simulink model "RobotStepID"  (R2022b)
settings: Solver=VariableStepAuto  StartTime=0.0  StopTime=10.0  RelTol=1e-3
values from neighbouring files (symbols this model uses):
  kPhi = 3.3*12.5    (= 41.25)    [demo1_avgVa_Identification.m]    (also in robotContVars.mat; robot_continuous_vars_workspace.m)
  kV = 0*0.51*12.5    (= 0)    [demo1_avgVa_Identification.m]    (also in robotContVars.mat = 6.375; robot_continuous_vars_workspace.m = 6.375)
  om_nPhi = 1*12.5    (= 12.5)    [demo1_avgVa_Identification.m]    (also in robotContVars.mat; robot_continuous_vars_workspace.m)
  om_nV = 1*12.5    (= 12.5)    [demo1_avgVa_Identification.m]    (also in robotContVars.mat; robot_continuous_vars_workspace.m)
  setaPhi = 1.55    [demo1_avgVa_Identification.m]    (also in robotContVars.mat; robot_continuous_vars_workspace.m)
  setaV = 1.33    [demo1_avgVa_Identification.m]    (also in robotContVars.mat; robot_continuous_vars_workspace.m)
settings Model: Creator=Charles A Vath  LastModifiedBy=Charles A Vath

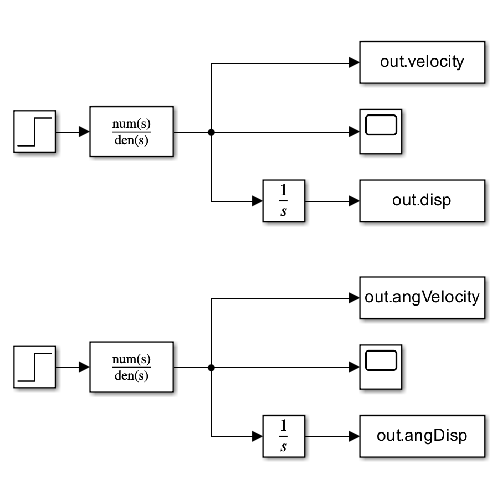
[thumbnail: Simulink's stored preview of the top-level diagram]
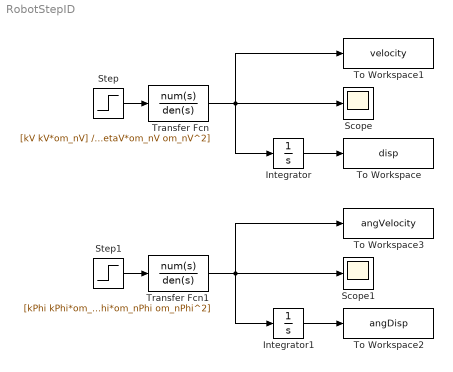
== system RobotStepID ==
  Integrator : Integrator
  Integrator1 : Integrator
  Scope : Scope
  Scope1 : Scope
  Step : Step  SampleTime=0
  Step1 : Step  SampleTime=0
  To Workspace : ToWorkspace  VariableName=disp  SaveFormat=Timeseries  SampleTime=-1
  To Workspace1 : ToWorkspace  VariableName=velocity  SaveFormat=Timeseries  SampleTime=-1
  To Workspace2 : ToWorkspace  VariableName=angDisp  SaveFormat=Timeseries  SampleTime=-1
  To Workspace3 : ToWorkspace  VariableName=angVelocity  SaveFormat=Timeseries  SampleTime=-1
  Transfer Fcn : TransferFcn  Numerator=[kV kV*om_nV]  Denominator=[1 2*setaV*om_nV om_nV^2]
  Transfer Fcn1 : TransferFcn  Numerator=[kPhi kPhi*om_nPhi]  Denominator=[1 2*setaPhi*om_nPhi om_nPhi^2]
  wires:
  Integrator/1 -> To Workspace/1
  Transfer Fcn/1 -> Integrator/1, To Workspace1/1, Scope/1
  Step/1 -> Transfer Fcn/1
  Integrator1/1 -> To Workspace2/1
  Transfer Fcn1/1 -> Integrator1/1, To Workspace3/1, Scope1/1
  Step1/1 -> Transfer Fcn1/1
